simulink model "sigma_delta_1er_ordre_z"  (Simulink 8.6)
settings: Solver=FixedStepAuto  StartTime=0.0  StopTime=t_sim  FixedStep=1/fck  RelTol=1e-3
values from neighbouring files (symbols this model uses):
  fck = 1000000    [main_sigma_delta.m]
  noise = 1e4/fck^2    (= 1e-08)    [main_sigma_delta.m]
  tau = 1/(2*pi*fc)    (= 0.0159154943092)    [main_sigma_delta.m]
libraries: simulink x1
settings Model: Creator=mailly  LastModifiedBy=mailly
settings OptimizationCC: ExpressionDepthLimit=128  InitFltsAndDblsToZero=on
settings DebuggingCC: SaveWithParameterizedLinksMsg=none  SignalResolutionControl=TryResolveAllWithWarning  MultiTaskDSMMsg=warning  MultiTaskCondExecSysMsg=none  FcnCallInpInsideContextMsg=UseLocalSettings  StateNameClashWarn=none  StrictBusMsg=None
settings GRTTargetCC: TargetFcnLib=ansi_tfl_tmw.mat  GeneratePreprocessorConditionals=Use local settings

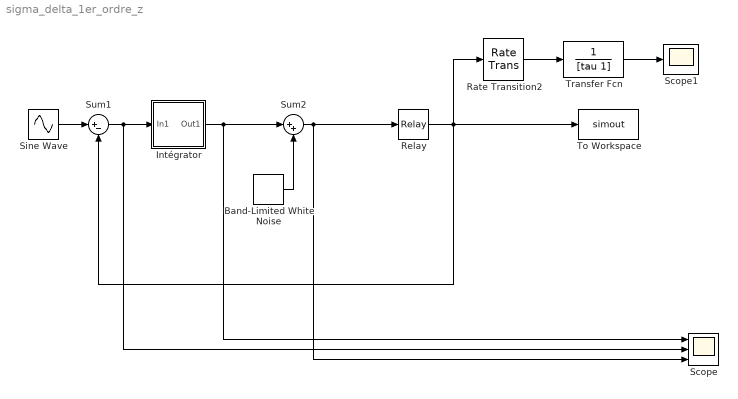
== system sigma_delta_1er_ordre_z ==
  Band-Limited White Noise : simulink/Sources/Band-Limited White Noise  Cov=[noise]  Ts=1/fck  seed=[23341]
  Intégrator : Subsystem
  Rate Transition2 : RateTransition
  Relay : Relay  OnSwitchValue=0  OffSwitchValue=0  OffOutputValue=-1  SampleTime=1/fck
  Scope : Scope  NumInputPorts=3
  Scope1 : Scope
  Sine Wave : Sin  Amplitude=0.5  Frequency=2*pi*10  SampleTime=1/fck
  Sum1 : Sum  Inputs=|+-
  Sum2 : Sum  Inputs=|++
  To Workspace : ToWorkspace  VariableName=simout  SampleTime=1/fck
      settings: MaxDataPoints=fck
  Transfer Fcn : TransferFcn  Denominator=[tau 1]
  wires:
  Sine Wave/1 -> Sum1/1
  Sum1/1 -> Scope/2, Intégrator/1(In1)
  Relay/1 -> To Workspace/1, Rate Transition2/1, Sum1/2
  Band-Limited White Noise/1 -> Sum2/2
  Sum2/1 -> Scope/3, Relay/1
  Transfer Fcn/1 -> Scope1/1
  Rate Transition2/1 -> Transfer Fcn/1
  Intégrator/1(Out1) -> Sum2/1, Scope/1

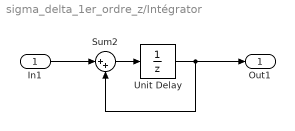
== system sigma_delta_1er_ordre_z/Intégrator ==
  In1 : Inport
  Sum2 : Sum  Inputs=|++
  Unit Delay : UnitDelay  SampleTime=1/fck
  Out1 : Outport
  wires:
  In1/1 -> Sum2/1
  Sum2/1 -> Unit Delay/1
  Unit Delay/1 -> Out1/1, Sum2/2
